simulink model "lab_part3"  (R2022a)
settings: Solver=ode45  StartTime=0.0  StopTime=3.0  RelTol=1e-3
values from neighbouring files (symbols this model uses):
  a = 2.5    [part3_plot.m]
  zeta = .6    (= 0.6)    [init.m]    (also in part3_plot.m)
settings Model: Creator=zhong  LastModifiedBy=zhong
settings DataIOCC: ReturnWorkspaceOutputs=off

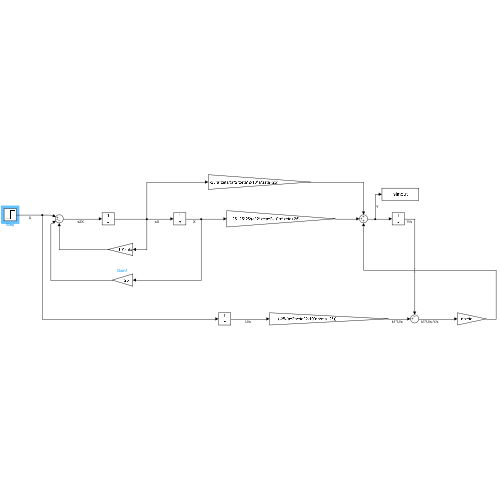
[thumbnail: Simulink's stored preview of the top-level diagram]
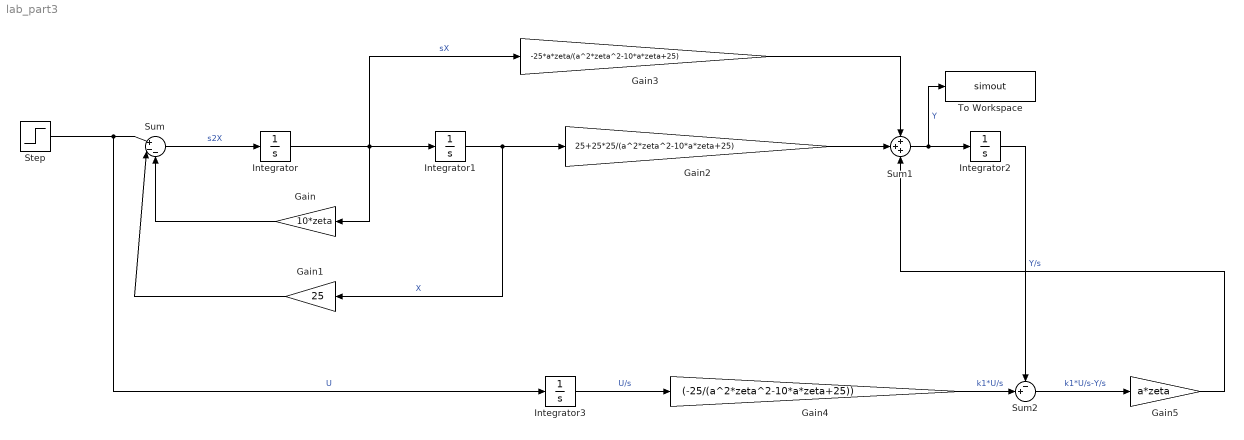
== system lab_part3 ==
  Gain : Gain  Gain=10*zeta
  Gain1 : Gain  Gain=25
  Gain2 : Gain  Gain=25+25*25/(a^2*zeta^2-10*a*zeta+25)
  Gain3 : Gain  Gain=-25*a*zeta/(a^2*zeta^2-10*a*zeta+25)
  Gain4 : Gain  Gain=(-25/(a^2*zeta^2-10*a*zeta+25))
  Gain5 : Gain  Gain=a*zeta
  Integrator{,1..3} (4 alike) : Integrator
  Step : Step  Time=0  SampleTime=0
  Sum : Sum  Inputs=|+--
  Sum1 : Sum  Inputs=+++
  Sum2 : Sum  Inputs=-+|
  To Workspace : ToWorkspace  VariableName=simout  SampleTime=-1
  wires:
  Sum/1 -> Integrator/1  "s2X"
  Integrator/1 -> Gain/1, Gain3/1, Integrator1/1  "sX"
  Integrator1/1 -> Gain1/1, Gain2/1  "X"
  Gain2/1 -> Sum1/2
  Gain3/1 -> Sum1/1
  Sum1/1 -> Integrator2/1, To Workspace/1  "Y"
  Gain/1 -> Sum/3
  Gain1/1 -> Sum/2
  Step/1 -> Integrator3/1, Sum/1  "U"
  Integrator3/1 -> Gain4/1  "U/s"
  Gain4/1 -> Sum2/2  "k1*U/s"
  Integrator2/1 -> Sum2/1  "Y/s"
  Sum2/1 -> Gain5/1  "k1*U/s-Y/s"
  Gain5/1 -> Sum1/3
